simulink model "FanModel_BJT"  (R2023a)
settings: Solver=ode4  StartTime=0.0  StopTime=0.1  FixedStep=0.00005  RelTol=1e-3
libraries: spsIGBTDiodeLib x4, spsDCVoltageSourceLib x2, spsDCMachineLib x1, sps_lib x1
settings Model: Creator=koush  LastModifiedBy=koush
settings SolverCC: ZeroCrossAlgorithm=Adaptive
settings DebuggingCC: IgnoredZcDiagnostic=none

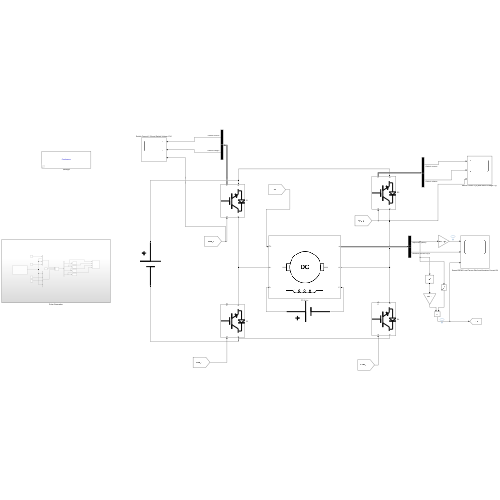
[thumbnail: Simulink's stored preview of the top-level diagram]
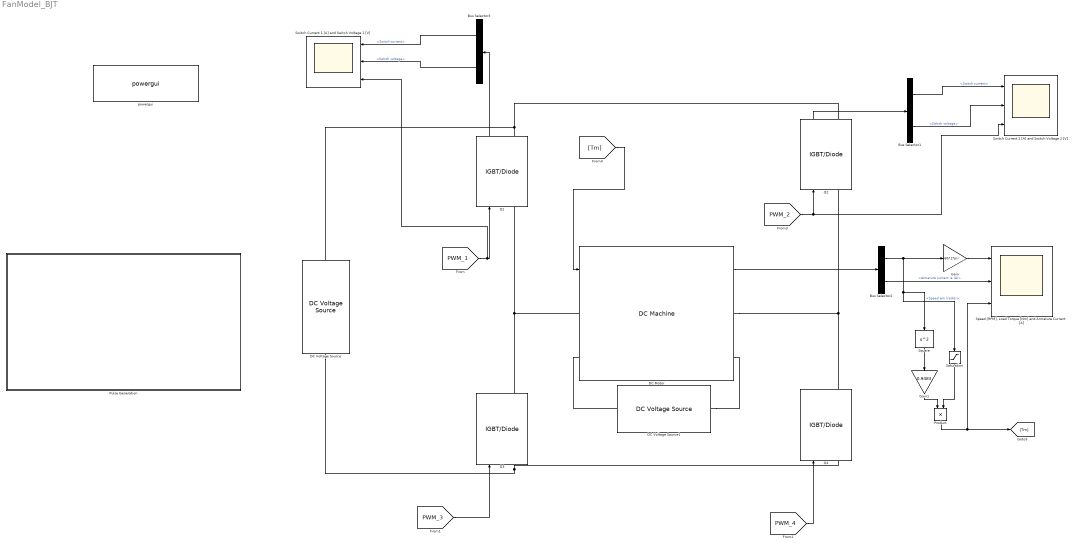
== system FanModel_BJT ==
  Bus Selector1 : BusSelector  OutputSignals=Switch current,Switch voltage
  Bus Selector2 : BusSelector  OutputSignals=Speed wm (rad/s),Armature current ia (A)
  Bus Selector3 : BusSelector  OutputSignals=Switch current,Switch voltage
  DC Motor : spsDCMachineLib/DC Machine  PresetModel=01: 5HP 240V 1750RPM Field:300V  MechanicalLoad=Torque TL  FieldType=Wound  ShowDetailedParameters=on  MeasurementBus=off  RLa=[2.581 0.028]  RLf=[281.2 156]  Laf=0.9483  MachineConstant=Torque constant (N.m/A)  Ke=1.8  Kt=1.8  J=0.02215  Bm=0.002953  Tf=0.5161  w0=1  Ifinit=1.06685633001422  TsPowergui=0  TsBlock=-1
  DC Voltage Source : spsDCVoltageSourceLib/DC Voltage Source  Amplitude=240  Measurements=Voltage
  DC Voltage Source1 : spsDCVoltageSourceLib/DC Voltage Source  Amplitude=300  Measurements=Voltage
  Gain : Gain  Gain=60/(2*pi)
  Gain1 : Gain  Gain=0.9483
  Product : Product
  Pulse Generation : Subsystem
  Q{1..4} (4 alike) : spsIGBTDiodeLib/IGBT//Diode  Ron=1e-3  Rs=1e5  Cs=inf  Measurements=on
  Saturation : Saturate
  "Speed [RPM], Load Torque [Nm] and Armature Current [A]" : Scope  NumInputPorts=3
  Square : Math  Operator=square
  Switch Current 1 [A] and Switch Voltage 1 [V] : Scope  NumInputPorts=3
  Switch Current 2 [A] and Switch Voltage 2 [V] : Scope  NumInputPorts=3
  powergui : sps_lib/powergui  Priority=1  SimulationMode=Continuous  SampleTime=50e-6  frequency=60  Iterations=50  frequencyindice=0  Pbase=100e6  ErrMax=1e-4  UnitsV=kV  UnitsW=MW  buscounter=0  FunctionMessages=off  echomessages=off  EnableUseOfTLC=off  CurrentSourceSwitches=off  DisableSnubberDevices=off  DisableRonSwitches=off  DisableVfSwitches=off  DisplayEquations=off  AutomaticDiscreteSolvers=off  SolverType=Tustin/Backward Euler (TBE)  Interpol=off  ExternalGateDelay=off  methode=off  Ts=100  x0status=blocks  SPID=on  SwTol=0  HookPort=off  NonlinearTolerance=1e-4  nMaxIteration=100  ContinueOnMaxIteration=off  RestoreLinks=warning  ResistiveCurrentMeasurement=off  Frange=[0:2:500]  Ylog=off  Xlog=on  ShowGrid=off  save=off  variable=ZData  structure=0  ZoomFFT=off  StartTime=0.0  cycles=1  DisplayStyle=1  fundamental=60  FreqAxis=off  MaxFrequency=1000  frequencyindicesteady=1  RmsSteady=1  display=off
  wires:
  [PWM_4] -> Q4/1
  [PWM_2] -> Q2/1, Switch Current 2 [A] and Switch Voltage 2 [V]/3
  [PWM_1] -> Switch Current 1 [A] and Switch Voltage 1 [V]/3, Q1/1
  [PWM_3] -> Q3/1
  [Tm] -> DC Motor/1
  Q2/1 -> Bus Selector1/1
  Bus Selector1/1 -> Switch Current 2 [A] and Switch Voltage 2 [V]/1  "<Switch current>"
  DC Motor/1 -> Bus Selector2/1
  Bus Selector2/1 -> Saturation/1, Square/1, Gain/1  "<Speed wm (rad/s)>"
  Gain/1 -> "Speed [RPM], Load Torque [Nm] and Armature Current [A]"/1
  Bus Selector2/2 -> "Speed [RPM], Load Torque [Nm] and Armature Current [A]"/2  "<Armature current ia (A)>"
  Square/1 -> Gain1/1
  Gain1/1 -> Product/1
  Saturation/1 -> Product/2
  Product/1 -> "Speed [RPM], Load Torque [Nm] and Armature Current [A]"/3, [Tm]
  Bus Selector1/2 -> Switch Current 2 [A] and Switch Voltage 2 [V]/2  "<Switch voltage>"
  Q1/1 -> Bus Selector3/1
  Bus Selector3/1 -> Switch Current 1 [A] and Switch Voltage 1 [V]/1  "<Switch current>"
  Bus Selector3/2 -> Switch Current 1 [A] and Switch Voltage 1 [V]/2  "<Switch voltage>"
  connections:
  DC Motor/LConn1 -- Q1/LConn1 -- Q3/RConn1
  DC Voltage Source/LConn1 -- Q4/LConn1 -- Q3/LConn1
  DC Motor/RConn1 -- Q2/LConn1 -- Q4/RConn1
  DC Voltage Source/RConn1 -- Q1/RConn1 -- Q2/RConn1
  DC Voltage Source1/RConn1 -- DC Motor/LConn2
  DC Voltage Source1/LConn1 -- DC Motor/RConn2

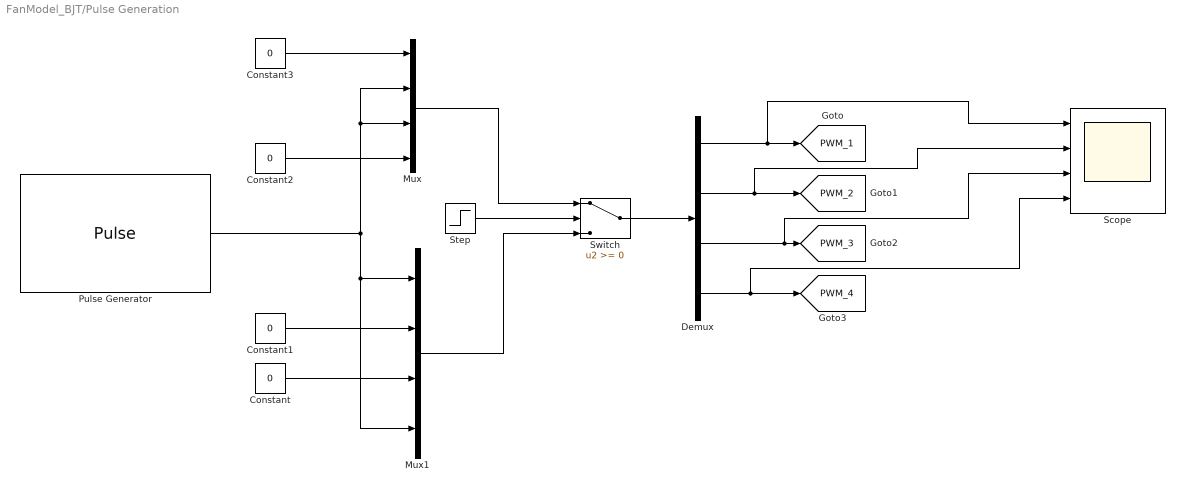
== system FanModel_BJT/Pulse Generation ==
  Constant{,1..3} (4 alike) : Constant  Value=0
  Demux : Demux
  Mux : Mux
  Mux1 : Mux
  Pulse Generator : DiscretePulseGenerator  PulseType=Time based  Amplitude=240  Period=0.002  PulseWidth=40
  Scope : Scope  NumInputPorts=4
  Step : Step  SampleTime=0
  Switch : Switch  SaturateOnIntegerOverflow=off  InputSameDT=off
  tag scope: PWM_1=global, PWM_2=global, PWM_3=global, PWM_4=global
  wires:
  Demux/1 -> Scope/1, [PWM_1]
  Demux/4 -> Scope/4, [PWM_4]
  Constant3/1 -> Mux/1
  Mux/1 -> Switch/1
  Constant/1 -> Mux1/3
  Step/1 -> Switch/2
  Constant1/1 -> Mux1/2
  Constant2/1 -> Mux/4
  Demux/2 -> Scope/2, [PWM_2]
  Demux/3 -> Scope/3, [PWM_3]
  Mux1/1 -> Switch/3
  Switch/1 -> Demux/1
  Pulse Generator/1 -> Mux1/4, Mux1/1, Mux/3, Mux/2
